simulink model "Foc_2024b"  (R2025a)
settings: Solver=FixedStepDiscrete  StartTime=0.0  StopTime=10.0  FixedStep=0.001  RelTol=1e-3
values from neighbouring files (symbols this model uses):
  cal_AdcMaxCountsHw = NoneSAR.Parameter    [Foc_2024b_LoadCalParameter.m]
  cal_AdcRefVoltHw = NoneSAR.Parameter    [Foc_2024b_LoadCalParameter.m]
  cal_AdcVoltMidHw = NoneSAR.Parameter    [Foc_2024b_LoadCalParameter.m]
  cal_bActHwMode = NoneSAR.Parameter    [Foc_2024b_LoadCalParameter.m]    (also in Foc_LoadCalParameter.m)
  cal_FullScaleCur = NoneSAR.Parameter    [Foc_2024b_LoadCalParameter.m]
  cal_GainAmpHw = NoneSAR.Parameter    [Foc_2024b_LoadCalParameter.m]
  cal_HwtDutyU = NoneSAR.Parameter    [Foc_2024b_LoadCalParameter.m]
  cal_HwtDutyV = NoneSAR.Parameter    [Foc_2024b_LoadCalParameter.m]
  cal_HwtDutyW = NoneSAR.Parameter    [Foc_2024b_LoadCalParameter.m]
  cal_HwtSector = NoneSAR.Parameter    [Foc_2024b_LoadCalParameter.m]
  cal_OhmRShuntHw = NoneSAR.Parameter    [Foc_2024b_LoadCalParameter.m]
  cal_s16Inductivity = NoneSAR.Parameter    [Foc_2024b_LoadCalParameter.m]    (also in Foc_LoadCalParameter.m)
  cal_s16LpfPllEst = NoneSAR.Parameter    [Foc_2024b_LoadCalParameter.m]    (also in Foc_LoadCalParameter.m)
  cal_s16LpfPllEstOpenLoop = NoneSAR.Parameter    [Foc_2024b_LoadCalParameter.m]    (also in Foc_LoadCalParameter.m)
  cal_s16MinSampleTime = NoneSAR.Parameter    [Foc_2024b_LoadCalParameter.m]    (also in Foc_LoadCalParameter.m)
  cal_s16OmegaGainEst = NoneSAR.Parameter    [Foc_2024b_LoadCalParameter.m]    (also in Foc_LoadCalParameter.m)
  cal_s16RPha = NoneSAR.Parameter    [Foc_2024b_LoadCalParameter.m]    (also in Foc_LoadCalParameter.m)
  cal_s16ThresholdPhaCurImplaisible = NoneSAR.Parameter    [Foc_2024b_LoadCalParameter.m]    (also in Foc_LoadCalParameter.m)
  cal_u8TiDebPhaCur = NoneSAR.Parameter    [Foc_2024b_LoadCalParameter.m]    (also in Foc_LoadCalParameter.m)
undefined symbols (not defined in the file or in its folder): AdcTriggerOffset, CCU6_T12PERIOD, CCU_PWM_PERIOD_TICKS_HALF, DCLINK_VOLTAGE_FACTOR, DesiredPwm_U, DesiredPwm_V, DesiredPwm_W, e_motorstate_t, e_running_dir_t, FOC_SVM_MAX, FOC_VD_VQ_MAX, FOC_VD_VQ_MAX_100, FOC_VD_VQ_MAX_95, FOC_VD_VQ_MAX_97, FOCLLD_CCU_PWM_PERIOD_TICKS_HALF, FOCLLD_SKIP_DEAD_TIME_THRESHOLD, MAX_DUTY, MIN_SAMPLE_TIME_DEFAULT, MODULATION_FLATBOTTOM, ONEBY_CURRENT_AMPLIFICATION, PhaseCurrentU, PhaseCurrentV, PhaseCurrentW, PwmShift_DutyLong, PwmShift_DutyMed, PwmShift_DutyShort, PwmShiftPtr_RiseLong, PwmShiftPtr_RiseMed, PwmShiftPtr_RiseShort, s16_EST_THETA_GAIN, s16_ONEBYSQR3, s16_SQR3OVER2, st_c_pi_Q_s16_outMax, st_c_pi_Q_s16_outMin, U8_INDUCTIVITY_FAC, VQ_MAX_TABLE_SIZE, VqMaxTable_100, VqMaxTable_95, VqMaxTable_97
libraries: simulink x16, hdlsllib x2
(part 6 of 6)

== system Foc_2024b/FieldOrientedControl/SetDutyCycle/PreCondition/SectorDetectionPart2/Sector_6_2/Sector2 ==
  s16Vv : Inport  OutDataTypeStr=int16
  s16Vw : Inport  Port=2  OutDataTypeStr=int16
  eMduMotCtrl : Inport  Port=3  OutDataTypeStr=Enum: auto
  Action Port : ActionPort
  Add : Sum  Inputs=+-
  Add1 : Sum
  Add2 : Sum
  Add3 : Sum
  Constant : Constant  Value=3
  Constant1 : Constant  Value=MODULATION_FLATBOTTOM
  Constant2 : Constant  Value=0  OutDataTypeStr=int16
  Constant3 : Constant  Value=FOC_SVM_MAX
  Constant4 : Constant  Value=2  OutDataTypeStr=int16
  Divide : Product  Inputs=*/
  Relational Operator : RelationalOperator  Operator===  OutDataTypeStr=boolean  RndMeth=Simplest  InputSameDT=off
  Switch : Switch  Criteria=u2 ~= 0  SaturateOnIntegerOverflow=off  InputSameDT=off
  Switch1 : Switch  Criteria=u2 ~= 0  SaturateOnIntegerOverflow=off  InputSameDT=off
  stSvmDutyW : Outport
  u8SvmSector : Outport  Port=2  OutDataTypeStr=uint8
  stSvmDutyU : Outport  Port=3
  stSvmDutyV : Outport  Port=4
  wires:
  Divide/1 -> Switch/3
  s16Vw/1 -> [s16Vw]
  eMduMotCtrl/1 -> Relational Operator/1
  [s16_svm_dutycycle_b] -> Add3/1
  [s16Vv] -> Add1/2
  s16Vv/1 -> [s16Vv]
  Constant/1 -> u8SvmSector/1
  Add1/1 -> Add/2
  Constant3/1 -> Add/1
  [s16Vw] -> Add1/1
  [s16Vv] -> Add3/2
  Add/1 -> Divide/1
  Add3/1 -> stSvmDutyU/1
  Constant4/1 -> Divide/2
  Constant1/1 -> Relational Operator/2
  [s16_svm_dutycycle_c] -> Add2/1
  [s16Vw] -> Add2/2
  Constant2/1 -> Switch/1
  Relational Operator/1 -> Switch/2, Switch1/2
  [s16Vw] -> Switch1/1
  Add2/1 -> Switch1/3
  Switch/1 -> stSvmDutyW/1, [s16_svm_dutycycle_c]
  Switch1/1 -> stSvmDutyV/1, [s16_svm_dutycycle_b]

== system Foc_2024b/FieldOrientedControl/SetDutyCycle/PreCondition/SectorDetectionPart2/Sector_6_2/Sector6 ==
  s16Vv : Inport  OutDataTypeStr=int16
  s16Vw : Inport  Port=2  OutDataTypeStr=int16
  eMduMotCtrl : Inport  Port=3  OutDataTypeStr=Enum: auto
  Action Port : ActionPort
  Add : Sum  Inputs=+-
  Add1 : Sum
  Add2 : Sum
  Add3 : Sum
  Constant : Constant  Value=3
  Constant1 : Constant  Value=MODULATION_FLATBOTTOM
  Constant2 : Constant  Value=0  OutDataTypeStr=int16
  Constant3 : Constant  Value=FOC_SVM_MAX
  Constant4 : Constant  Value=2  OutDataTypeStr=int16
  Divide : Product  Inputs=*/
  Relational Operator : RelationalOperator  Operator===  OutDataTypeStr=boolean  RndMeth=Simplest  InputSameDT=off
  Switch : Switch  Criteria=u2 ~= 0  SaturateOnIntegerOverflow=off  InputSameDT=off
  Switch1 : Switch  Criteria=u2 ~= 0  SaturateOnIntegerOverflow=off  InputSameDT=off
  stSvmDutyW : Outport
  u8SvmSector : Outport  Port=2  OutDataTypeStr=uint8
  stSvmDutyU : Outport  Port=3
  stSvmDutyV : Outport  Port=4
  wires:
  Switch/1 -> stSvmDutyW/1, [s16_svm_dutycycle_c]
  s16Vw/1 -> [s16Vw]
  [s16_svm_dutycycle_b] -> Add3/1
  [s16Vv] -> Add1/2
  Constant/1 -> u8SvmSector/1
  Constant3/1 -> Add/1
  [s16Vw] -> Add1/1
  s16Vv/1 -> [s16Vv]
  [s16Vv] -> Add3/2
  Add1/1 -> Add/2
  Add3/1 -> stSvmDutyU/1
  Add/1 -> Divide/1
  Constant4/1 -> Divide/2
  eMduMotCtrl/1 -> Relational Operator/1
  Constant1/1 -> Relational Operator/2
  [s16_svm_dutycycle_c] -> Add2/1
  [s16Vw] -> Add2/2
  Constant2/1 -> Switch/1
  Divide/1 -> Switch/3
  Relational Operator/1 -> Switch1/2, Switch/2
  [s16Vw] -> Switch1/1
  Add2/1 -> Switch1/3
  Switch1/1 -> stSvmDutyV/1, [s16_svm_dutycycle_b]

== system Foc_2024b/FieldOrientedControl/CurrentControl/MOTOR_STATE_CLOSED_LOOP/ PiCtrl_Calc/ CalcVqMax/GetVqMax/GetVqMax ==
  Vd : Inport  OutDataTypeStr=fixdt(1,16,15)
  Index : Inport  Port=2
  VQ_MAX_TABLE_SIZE : Inport  Port=3
  VqMaxTable : Inport  Port=4
  Constant1 : Constant  Value=2
  Relational Operator : RelationalOperator  Operator=<=  OutDataTypeStr=boolean  RndMeth=Simplest  InputSameDT=off
  Subtract : Sum  Inputs=+-
  Switch : Switch  Criteria=u2 ~= 0  SaturateOnIntegerOverflow=off  InputSameDT=off
  VaMax_ValidIndex : Subsystem
  VqMax_InvalidIndex : Subsystem
  VqMax : Outport
  wires:
  [VQ_MAX_TABLE_SIZE] -> Subtract/1
  Constant1/1 -> Subtract/2
  Subtract/1 -> Relational Operator/2
  [Index] -> Relational Operator/1
  Relational Operator/1 -> Switch/2
  Vd/1 -> VaMax_ValidIndex/1(Vd)
  [VQ_MAX_TABLE_SIZE] -> VaMax_ValidIndex/3(Index)
  [VQ_MAX_TABLE_SIZE] -> VqMax_InvalidIndex/2(VQ_MAX_TABLE_SIZE)
  [VqMaxTable] -> VqMax_InvalidIndex/1(VqMaxTable)
  [VqMaxTable] -> VaMax_ValidIndex/2(VqMaxTable)
  Switch/1 -> VqMax/1
  VqMaxTable/1 -> [VqMaxTable]
  VQ_MAX_TABLE_SIZE/1 -> [VQ_MAX_TABLE_SIZE]
  Index/1 -> [Index]
  VaMax_ValidIndex/1(VqMax) -> Switch/1
  VqMax_InvalidIndex/1(VqMax) -> Switch/3

== system Foc_2024b/FieldOrientedControl/CurrentControl/MOTOR_STATE_CLOSED_LOOP/ PiCtrl_Calc/ CalcVqMax/GetVqMax/Index ==
  Vd_In : Inport  OutDataTypeStr=fixdt(1,16,15)
  Abs : Abs  SaturateOnIntegerOverflow=off
  Constant : Constant  Value=0  OutDataTypeStr=uint8
  Constant1 : Constant  Value=30  OutDataTypeStr=uint8
  Gain : Gain  Gain=1/1024  OutDataTypeStr=int16
  Saturation Dynamic : simulink/Discontinuities/Saturation Dynamic  OutMin=[]  OutMax=[]  OutDataTypeStr=Inherit: Same as second input  OutDataType=fixdt(1, 16)  OutScaling=2^-10  DoSatur=off
  Index : Outport
  Vd : Outport  Port=2
  wires:
  Vd_In/1 -> Abs/1
  Abs/1 -> Vd/1, Gain/1  "Vd"
  Constant1/1 -> Saturation Dynamic/1
  Gain/1 -> Saturation Dynamic/2
  Constant/1 -> Saturation Dynamic/3
  Saturation Dynamic/1 -> Index/1

== system Foc_2024b/FieldOrientedControl/CurrentControl/MOTOR_STATE_CLOSED_LOOP/ PiCtrl_Calc/ CalcVqMax/GetVqMax/GetVqMax/VaMax_ValidIndex ==
  Vd : Inport
  VqMaxTable : Inport  Port=2
  Index : Inport  Port=3
  Add : Sum  Inputs=+-
  Add1 : Sum  Inputs=+-
  Constant : Constant
  Constant1 : Constant
  Constant3 : Constant  Value=1024  OutDataTypeStr=int16
  Data Type Conversion : DataTypeConversion  OutDataTypeStr=int16  SaturateOnIntegerOverflow=off  RndMeth=Floor
  Gain : Gain  Gain=32  OutDataTypeStr=int16
  Mod : Math  Operator=mod
  Q_Mul_s16s16_s16 : Subsystem
  Selector : Selector  IndexMode=Zero-based  InputPortWidth=VQ_MAX_TABLE_SIZE  IndexOptions=Index vector (port)  Indices=[1 3]  OutputSizes=1
  Selector1 : Selector  IndexMode=Zero-based  InputPortWidth=VQ_MAX_TABLE_SIZE  IndexOptions=Index vector (port)  Indices=[1 3]  OutputSizes=1
  Subtract1 : Sum  Inputs=+-
  VqMax : Outport
  wires:
  Constant1/1 -> Add1/2
  Vd/1 -> Data Type Conversion/1
  Index/1 -> Add1/1, Add/1
  Constant/1 -> Add/2
  Data Type Conversion/1 -> Mod/1
  VqMaxTable/1 -> Selector1/1, Selector/1
  Constant3/1 -> Mod/2
  Add1/1 -> Selector/2
  Add/1 -> Selector1/2
  Mod/1 -> Gain/1
  Selector/1 -> Subtract1/1, Q_Mul_s16s16_s16/1(VqMaxTable[index])  "VqMaxTable[index]"
  Selector1/1 -> Q_Mul_s16s16_s16/2(VqMaxTable[index+1])  "VqMaxTable[index+1]"
  [VdMod] -> Q_Mul_s16s16_s16/3(VqMod)
  Gain/1 -> [VdMod]
  Q_Mul_s16s16_s16/1(Step) -> Subtract1/2
  Subtract1/1 -> VqMax/1

== system Foc_2024b/FieldOrientedControl/CurrentControl/MOTOR_STATE_CLOSED_LOOP/ PiCtrl_Calc/ CalcVqMax/GetVqMax/GetVqMax/VqMax_InvalidIndex ==
  VqMaxTable : Inport
  VQ_MAX_TABLE_SIZE : Inport  Port=2
  Constant3 : Constant
  Selector : Selector  IndexMode=Zero-based  InputPortWidth=VQ_MAX_TABLE_SIZE  IndexOptions=Index vector (port)  Indices=[1 3]  OutputSizes=1
  Subtract1 : Sum  Inputs=+-
  VqMax : Outport
  wires:
  VQ_MAX_TABLE_SIZE/1 -> Subtract1/1
  Constant3/1 -> Subtract1/2
  VqMaxTable/1 -> Selector/1
  Subtract1/1 -> Selector/2
  Selector/1 -> VqMax/1

== system Foc_2024b/FieldOrientedControl/CurrentControl/MOTOR_STATE_CLOSED_LOOP/ PiCtrl_Calc/ CalcVqMax/GetVqMax/GetVqMax/VaMax_ValidIndex/Q_Mul_s16s16_s16 ==
  VqMaxTable[index] : Inport
  VqMaxTable[index+1] : Inport  Port=2
  VqMod : Inport  Port=3
  Data Type Conversion : DataTypeConversion  OutDataTypeStr=int16  SaturateOnIntegerOverflow=off  RndMeth=Floor
  Product : Product
  Saturation : Saturate  UpperLimit=32767  LowerLimit=-32768
  Shift Arithmetic : ArithShift  BitShiftNumber=15  BitShiftDirection=Right
  Subtract2 : Sum  Inputs=+-
  Step : Outport
  wires:
  Shift Arithmetic/1 -> Saturation/1
  VqMaxTable[index]/1 -> Subtract2/1
  VqMaxTable[index+1]/1 -> Subtract2/2
  VqMod/1 -> Product/2
  Subtract2/1 -> Product/1  "delta"
  Product/1 -> Shift Arithmetic/1
  Saturation/1 -> Data Type Conversion/1
  Data Type Conversion/1 -> Step/1
